simulink model "Model_lab2"  (R2020b)
settings: Solver=ode1  StartTime=0.0  StopTime=simul_t  RelTol=1e-3
undefined symbols (not defined in the file): du, G, Kt, M, Omega_0, U_0
settings Model: Creator=lucas  LastModifiedBy=alexa

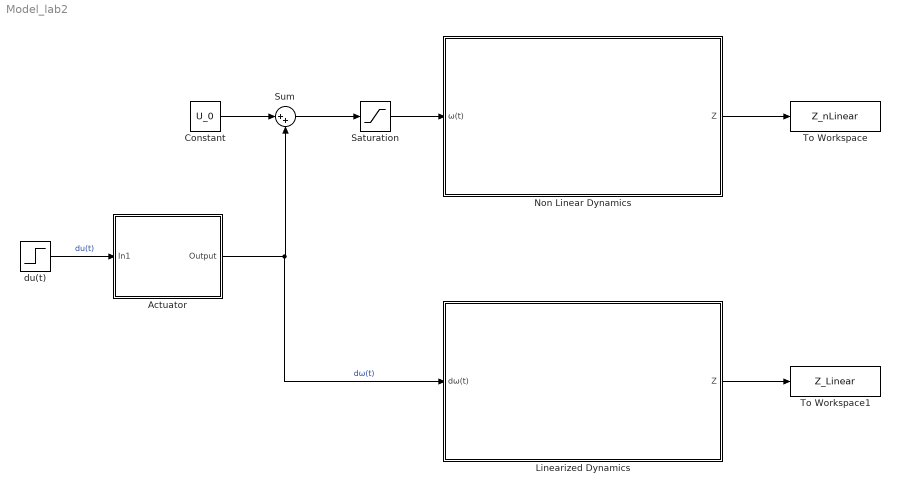
== system Model_lab2 ==
  Actuator : Subsystem
  Constant : Constant  Value=U_0
  Linearized Dynamics : Subsystem
  Non Linear Dynamics : Subsystem
  Saturation : Saturate  UpperLimit=3* Omega_0  LowerLimit=0
  Sum : Sum  Inputs=|++
  To Workspace : ToWorkspace  VariableName=Z_nLinear  SaveFormat=Structure With Time  SampleTime=-1
  To Workspace1 : ToWorkspace  VariableName=Z_Linear  SaveFormat=Structure With Time  SampleTime=-1
  du(t) : Step  Time=0  After=du  SampleTime=1
  wires:
  du(t)/1 -> Actuator/1(In1)  "du(t)"
  Non Linear Dynamics/1(Z) -> To Workspace/1
  Saturation/1 -> Non Linear Dynamics/1(ω(t))
  Actuator/1(Output) -> Linearized Dynamics/1(dω(t)), Sum/2  "dω(t)"
  Sum/1 -> Saturation/1
  Constant/1 -> Sum/1
  Linearized Dynamics/1(Z) -> To Workspace1/1

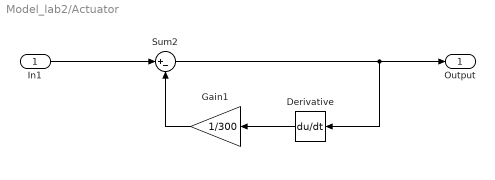
== system Model_lab2/Actuator ==
  In1 : Inport
  Derivative : Derivative
  Gain1 : Gain  Gain=1/300
  Sum2 : Sum  Inputs=|+-
  Output : Outport
  wires:
  In1/1 -> Sum2/1
  Sum2/1 -> Output/1, Derivative/1
  Derivative/1 -> Gain1/1
  Gain1/1 -> Sum2/2

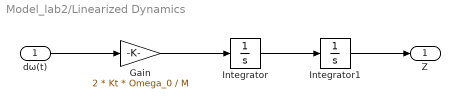
== system Model_lab2/Linearized Dynamics ==
  dω(t) : Inport
  Gain : Gain  Gain=2 * Kt * Omega_0 / M
  Integrator : Integrator
  Integrator1 : Integrator
  Z : Outport
  wires:
  dω(t)/1 -> Gain/1
  Integrator/1 -> Integrator1/1
  Gain/1 -> Integrator/1
  Integrator1/1 -> Z/1

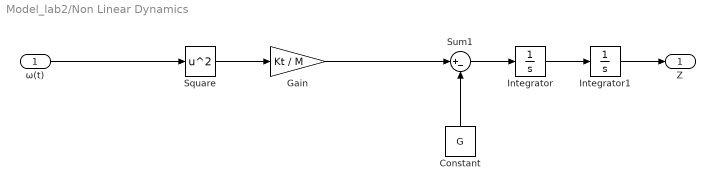
== system Model_lab2/Non Linear Dynamics ==
  ω(t) : Inport
  Constant : Constant  Value=G
  Gain : Gain  Gain=Kt / M
  Integrator : Integrator
  Integrator1 : Integrator
  Square : Math  Operator=square  OutputSignalType=real  SaturateOnIntegerOverflow=on
  Sum1 : Sum  Inputs=|+-
  Z : Outport
  wires:
  Square/1 -> Gain/1
  Gain/1 -> Sum1/1
  Integrator/1 -> Integrator1/1
  Sum1/1 -> Integrator/1
  Integrator1/1 -> Z/1
  ω(t)/1 -> Square/1
  Constant/1 -> Sum1/2
